simulink model "ddx"  (R2017b)
settings: Solver=FixedStepAuto  StartTime=0.0  StopTime=10.0  FixedStep=0.05  RelTol=1e-3
values from neighbouring files (symbols this model uses):
  dtheta0 = 0    [Simulation_based_test.m]
  dx0 = 0    [Simulation_based_test.m]
  g = 9.81    [Simulation_based_test.m]    (also in cart_pole.m; draft.m; dynamics.m; inv_pend.m = 9.8)
  l = length(max_order)    [MinCoverSOS.m]    (also in Simulation_based_test.m = 1; cart_pole.m = 1; draft.m = 1; dynamics.m = 1)
  m1 = 2.0    (= 2)    [Simulation_based_test.m]    (also in cart_pole.m; draft.m; dynamics.m; t1.mat)
  m2 = 0.5    [Simulation_based_test.m]    (also in cart_pole.m; draft.m; dynamics.m; t1.mat)
  theta0 = equilibrium_x(3) - 0.4    [Simulation_based_test.m]
  x0 = equilibrium_x(1) - 0.4    [Simulation_based_test.m]
settings Model: Creator=root  LastModifiedBy=root

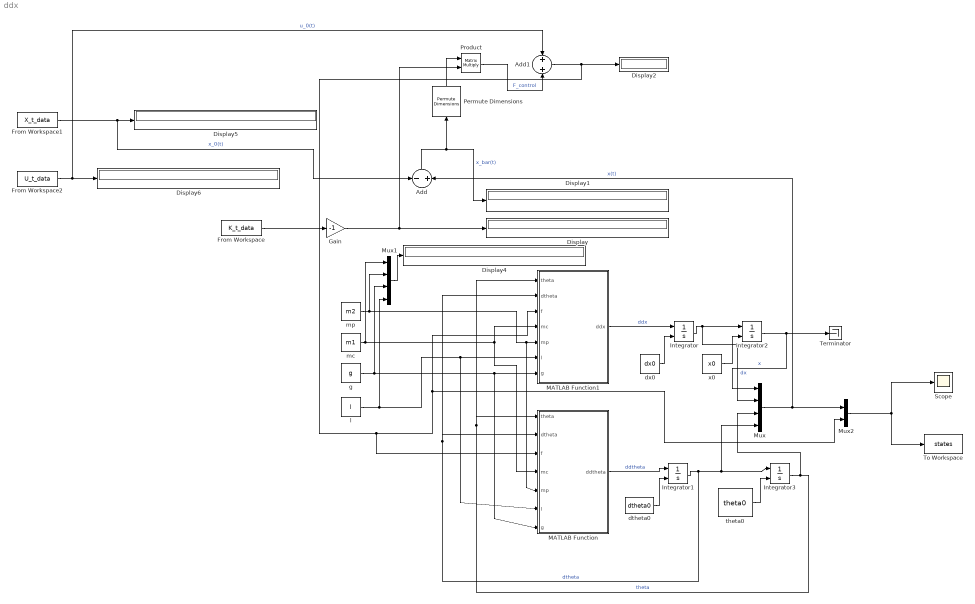
== system ddx ==
  Add : Sum  Inputs=-+
  Add1 : Sum
  Display{,1..2,4..6} (6 alike) : Display
  From Workspace : FromWorkspace  VariableName=K_t_data  SampleTime=0
  From Workspace1 : FromWorkspace  VariableName=X_t_data  SampleTime=0
  From Workspace2 : FromWorkspace  VariableName=U_t_data  SampleTime=0
  Gain : Gain  Gain=-1
  Integrator{,1..3} (4 alike) : Integrator  InitialConditionSource=external
  MATLAB Function : MATLAB Function  TreatAsAtomicUnit=on
  MATLAB Function1 : MATLAB Function  TreatAsAtomicUnit=on
  Mux : Mux
  Mux1 : Mux
  Mux2 : Mux  Inputs=2
  Permute Dimensions : PermuteDimensions
  Product : Product  Multiplication=Matrix(*)
  Scope : Scope
  Terminator : Terminator
  To Workspace : ToWorkspace  VariableName=states  SaveFormat=Timeseries  SampleTime=-1
  dtheta0 : Constant  Value=dtheta0
  dx0 : Constant  Value=dx0
  g : Constant  Value=g
  l : Constant  Value=l
  mc : Constant  Value=m1
  mp : Constant  Value=m2
  theta0 : Constant  Value=theta0
  x0 : Constant  Value=x0
  wires:
  MATLAB Function1/1(ddx) -> Integrator/1  "ddx"
  MATLAB Function/1(ddtheta) -> Integrator1/1  "ddtheta"
  Integrator/1 -> Mux/2, Integrator2/1  "dx"
  Integrator1/1 -> Mux/4, Integrator3/1, MATLAB Function/2(dtheta), MATLAB Function1/2(dtheta)  "dtheta"
  Integrator2/1 -> Mux/1, Terminator/1  "x"
  Integrator3/1 -> Mux/3, MATLAB Function1/1(theta), MATLAB Function/1(theta)  "theta"
  g/1 -> Mux1/3, MATLAB Function/7(g), MATLAB Function1/7(g)
  mc/1 -> Mux1/1, MATLAB Function/4(mc), MATLAB Function1/4(mc)
  mp/1 -> Mux1/2, MATLAB Function/5(mp), MATLAB Function1/5(mp)
  l/1 -> Mux1/4, MATLAB Function1/6(l), MATLAB Function/6(l)
  x0/1 -> Integrator2/2
  dx0/1 -> Integrator/2
  dtheta0/1 -> Integrator1/2
  theta0/1 -> Integrator3/2
  Mux/1 -> Add/2, Mux2/1  "x(t)"
  From Workspace/1 -> Gain/1
  Permute Dimensions/1 -> Product/1
  Add/1 -> Display1/1, Permute Dimensions/1  "x_bar(t)"
  Mux1/1 -> Display4/1
  From Workspace1/1 -> Add/1, Display5/1  "x_0(t)"
  From Workspace2/1 -> Add1/1, Display6/1  "u_0(t)"
  Gain/1 -> Display/1, Product/2
  Product/1 -> Add1/2  "F_control"
  Add1/1 -> MATLAB Function/3(f), Mux2/2, MATLAB Function1/3(f), Display2/1
  ? -> ?  "x(t)"
  Mux2/1 -> To Workspace/1, Scope/1

== matlab function ddx/MATLAB Function1 ==
  data: theta input; ddx output; dtheta input; f input; mc input; mp input; l input; g input
function ddx = ddx(theta, dtheta, f, mc, mp, l, g)

item1 = mc + mp * sin(theta)^2;
item2 = mp * sin(theta) * (l * dtheta^2 + g * cos(theta));
ddx = 1/item1 * (f + item2);

end

== matlab function ddx/MATLAB Function ==
  data: theta input; ddtheta output; dtheta input; f input; mc input; mp input; l input; g input
function ddtheta = ddtheta(theta, dtheta, f, mc, mp, l, g)

item1 = l * (mc + mp * sin(theta)^2);
item2 = mp * l * dtheta^2 * cos(theta) * sin(theta);
item3 = (mc + mp) * g * sin(theta);

ddtheta = 1/item1 * (-f*cos(theta) - item2 - item3 );

end
